simulink model "test_pid"  (R2013a)
settings: Solver=ode45  StartTime=0.0  StopTime=5  RelTol=1e-3
settings Model: Creator=rodrigo  LastModifiedBy=rodrigo

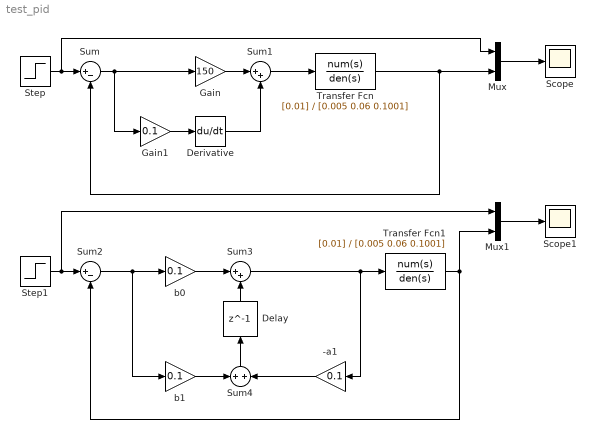
== system test_pid ==
  -a1 : Gain  Gain=0.1
  Delay : Delay  DelayLength=1
  Derivative : Derivative
  Gain : Gain  Gain=150
  Gain1 : Gain  Gain=0.1
  Mux : Mux  Inputs=2
  Mux1 : Mux  Inputs=2
  Scope : Scope
  Scope1 : Scope
  Step : Step  After=0.5  SampleTime=0
  Step1 : Step  After=0.5  SampleTime=0
  Sum : Sum  Inputs=|+-
  Sum1 : Sum  Inputs=|++
  Sum2 : Sum  Inputs=|+-
  Sum3 : Sum  Inputs=|++
  Sum4 : Sum  Inputs=+|+
  Transfer Fcn : TransferFcn  Numerator=[0.01]  Denominator=[0.005 0.06 0.1001]
  Transfer Fcn1 : TransferFcn  Numerator=[0.01]  Denominator=[0.005 0.06 0.1001]
  b0 : Gain  Gain=0.1
  b1 : Gain  Gain=0.1
  wires:
  Transfer Fcn/1 -> Sum/2, Mux/2
  Sum/1 -> Gain1/1, Gain/1
  Gain1/1 -> Derivative/1
  Derivative/1 -> Sum1/2
  Gain/1 -> Sum1/1
  Sum1/1 -> Transfer Fcn/1
  Step/1 -> Mux/1, Sum/1
  Mux/1 -> Scope/1
  Step1/1 -> Mux1/1, Sum2/1
  Mux1/1 -> Scope1/1
  Sum4/1 -> Delay/1
  b1/1 -> Sum4/1
  -a1/1 -> Sum4/2
  Sum2/1 -> b0/1, b1/1
  b0/1 -> Sum3/1
  Delay/1 -> Sum3/2
  Sum3/1 -> -a1/1, Transfer Fcn1/1
  Transfer Fcn1/1 -> Sum2/2, Mux1/2
